simulink model "lung_model"  (R2019b)
settings: Solver=VariableStepAuto  StartTime=0.0  StopTime=500  RelTol=1e-6  AbsTol=1e-3
values from neighbouring files (symbols this model uses):
  C = 0.02    [init_modell.m]
  Delta = 0.01    [init_modell.m]
  p0 = (V0-C*PEEP)/(-C)    (= -95)    [init_modell.m]
  PEEP = 5    [init_modell.m]
  Pinsp = 20    [init_modell.m]
  R = 50    [init_modell.m]
  Te = 2    [init_modell.m]
  Ti = 2    [init_modell.m]
  tt = 0:0.01:Ti    [init_modell.m]
  V0 = 2    [init_modell.m]
  yy = sin(2*pi/(Ti)*tt+pi*3/2)+1    [init_modell.m]
undefined symbols (not defined in the file or in its folder): DiscIntNeverNeededParam
libraries: simulink x2
settings Model: Creator=schauer  LastModifiedBy=schauer
settings SolverCC: ShapePreserveControl=EnableAll

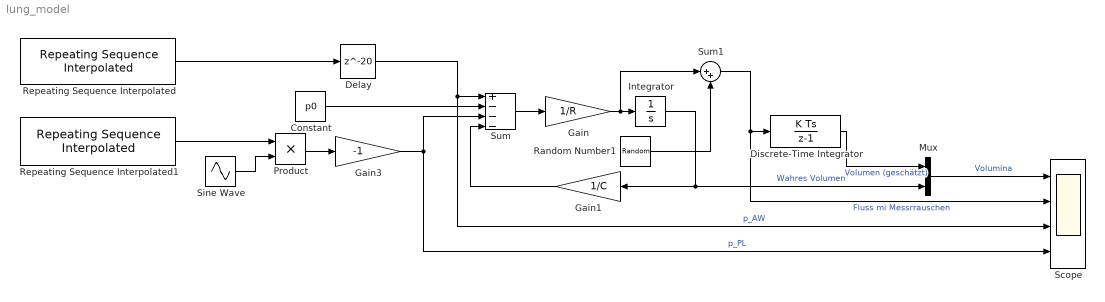
== system lung_model ==
  Constant : Constant  Value=p0
  Delay : Delay  DelayLength=20  InitialCondition=PEEP
  Discrete-Time Integrator : DiscreteIntegrator  gainval=1  SampleTime=Delta  ICPrevOutput=DiscIntNeverNeededParam  ICPrevScaledInput=DiscIntNeverNeededParam
  Gain : Gain  Gain=1/R
  Gain1 : Gain  Gain=1/C
  Gain3 : Gain  Gain=-1
  Integrator : Integrator  InitialCondition=V0
  Mux : Mux  Inputs=2
  Product : Product
  Random Number1 : RandomNumber  Variance=0.0001  SampleTime=Delta
  Repeating Sequence Interpolated : simulink/Sources/Repeating Sequence Interpolated  OutValues=[PEEP Pinsp Pinsp PEEP PEEP]'  TimeValues=[0 Ti/8 Ti Ti+0.01 Ti+Te].'  LookUpMeth=Interpolation-Use End Values  tsamp=Delta  OutMin=[]  OutMax=[]  OutDataTypeStr=double  OutputDataTypeScalingMode=double  OutDataType=fixdt(0,8)  OutScaling=2^-10
  Repeating Sequence Interpolated1 : simulink/Sources/Repeating Sequence Interpolated  OutValues=[yy 0]*5  TimeValues=[tt Ti+Te]  LookUpMeth=Interpolation-Use End Values  tsamp=Delta  OutMin=[]  OutMax=[]  OutDataTypeStr=double  OutputDataTypeScalingMode=double  OutDataType=fixdt(0,8)  OutScaling=2^-10
  Scope : Scope  NumInputPorts=4
  Sine Wave : Sin  Amplitude=0.5  Bias=0.5  Frequency=0.1*2*pi  SampleTime=0
  Sum : Sum  Inputs=+---
  Sum1 : Sum  Inputs=|++
  wires:
  Gain1/1 -> Sum/4
  Constant/1 -> Sum/2
  Sum/1 -> Gain/1
  Integrator/1 -> Mux/2, Gain1/1  "Wahres Volumen"
  Random Number1/1 -> Sum1/2
  Gain/1 -> Sum1/1, Integrator/1
  Mux/1 -> Scope/1  "Volumina"
  Sum1/1 -> Scope/2, Discrete-Time Integrator/1  "Fluss mi Messrrauschen"
  Delay/1 -> Scope/3, Sum/1  "p_AW"
  Gain3/1 -> Scope/4, Sum/3  "p_PL"
  Repeating Sequence Interpolated/1 -> Delay/1
  Product/1 -> Gain3/1
  Repeating Sequence Interpolated1/1 -> Product/1
  Sine Wave/1 -> Product/2
  Discrete-Time Integrator/1 -> Mux/1  "Volumen (geschätzt)"
